simulink model "lin_model_PI_MRAC_Sim_CASE1_L1"  (Simulink 7.7)
settings: Solver=ode45  StartTime=0.0  StopTime=TIME  RelTol=1e-3  AbsTol=1e-6
values from neighbouring files (symbols this model uses):
  Am = AA - BB*Kr    [lin_model_LQR.m]    (also in lin_model_PI_MRAC_CASE1.m = Ar-BB*Kr; lin_model_PI_MRAC_CASE1_L1.m = Ar-BB*Kr)
  Ar = Ar_cruise    [parameter.m]
  BB = B_cruise    [parameter.m]
  bm = -(CC*inv(Am))\eye(11)    [lin_model_PI_MRAC_CASE1.m]    (also in lin_model_PI_MRAC_CASE1_L1.m)
  gamma = rho*c_cr*a_cr*(r_cr)^4/Icr    (= 0.431761992187)    [beta_crS.m]    (also in heli_parameter.m = 5.40374741035; lin_model_PI_MRAC_CASE1.m = 1000000; lin_model_PI_MRAC_CASE1_L1.m = 10000; parameter.m = 5.40374741035)
  noise = 0.1    [lin_model_PI_MRAC_CASE1_L1.m]
  omega = 10    [lin_model_PI_MRAC_CASE1_L1.m]
  pulse = 1    [lin_model_PI_MRAC_CASE1_L1.m]
  tau = 0.01    [lin_model_PI_MRAC_CASE1_L1.m]
  Theta_a = AA-Ar    [parameter.m]
  theta_hat0 = eye(11)    [lin_model_PI_MRAC_CASE1.m]    (also in lin_model_PI_MRAC_CASE1_L1.m)
  unmodeled = 1    [lin_model_PI_MRAC_CASE1_L1.m]
  x0 = [0;0;0;0]    [beta_crS.m]    (also in flapping.m = []; flappingthrust.m = []; lin_flapping.m = []; lin_model_LQR.m = [3 3 3 0 0 0 0 0 0 0 0]')
  x_hat0 = x0    [lin_model_PI_MRAC_CASE1.m]    (also in lin_model_PI_MRAC_CASE1_L1.m)
undefined symbols (not defined in the file or in its folder): Kr
libraries: simulink x3, commnoisgen2 x1
settings Model: Creator=Li  LastModifiedBy=Li
settings DataIOCC: LimitDataPoints=off  SaveFormat=Structure
settings DebuggingCC: SolverPrmCheckMsg=none

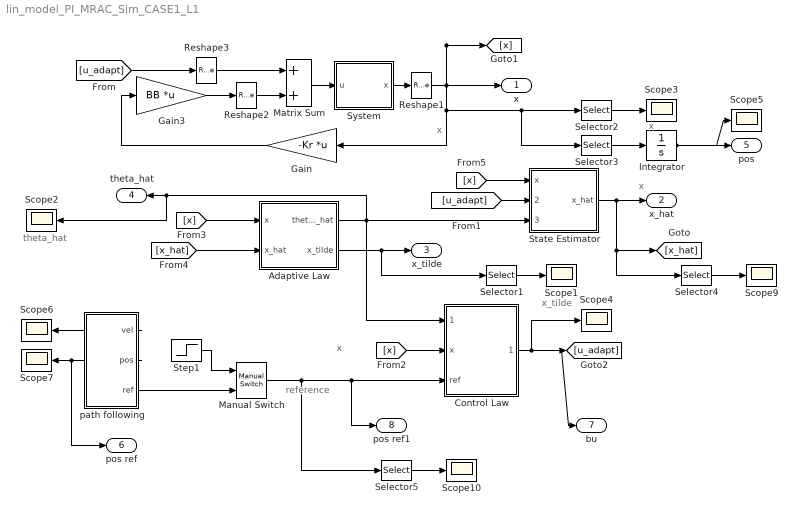
== system lin_model_PI_MRAC_Sim_CASE1_L1 ==
  note: x
  note: x
  note: reference
  note: theta_hat
  note: x_tilde
  note: x
  note: x
  Adaptive Law : Subsystem
  Control Law : Subsystem
  Gain : Gain  Gain=-Kr  Multiplication=Matrix(K*u) (u vector)
  Gain3 : Gain  Gain=BB  Multiplication=Matrix(K*u) (u vector)
  Integrator : Integrator
  Manual Switch : simulink/Signal Routing/Manual Switch  SystemSampleTime=-1  sw=0  action=0  varsize=off
  Matrix Sum : Sum
  Reshape1 : Reshape  OutputDimensionality=Column vector (2-D)
  Reshape2 : Reshape  OutputDimensionality=Column vector (2-D)
  Reshape3 : Reshape  OutputDimensionality=Column vector (2-D)
  Scope{1..7,9..10} (9 alike) : Scope
      Scope1 settings: TimeRange=3  YMin=-3e+007  YMax=2.5e+006
      Scope10 settings: TimeRange=10  YMin=-15  YMax=15  SaveName=ScopeData9
      Scope2 settings: TimeRange=20  YMin=-1  YMax=1
      Scope3 settings: TimeRange=10  YMin=-1400  YMax=0  SaveName=ScopeData2
      Scope4 settings: TimeRange=20  YMin=-150  YMax=300  SaveName=ScopeData3
      Scope5 settings: TimeRange=10  YMin=-3000  YMax=3000  SaveName=ScopeData4
      Scope6 settings: TimeRange=10  YMin=-3000  YMax=3000  SaveName=ScopeData5
      Scope7 settings: TimeRange=10  YMin=-3000  YMax=3000  SaveName=ScopeData6
      Scope9 settings: TimeRange=10  YMin=-15  YMax=17.5  SaveName=ScopeData8
  Selector1 : Selector  InputPortWidth=11  IndexOptions=Index vector (dialog)  Indices=[1 2 3 4 5]  OutputSizes=1
  Selector{2..5} (4 alike) : Selector  InputPortWidth=11  IndexOptions=Index vector (dialog)  Indices=[1 2 3]  OutputSizes=1
  State Estimator : Subsystem
  Step1 : Step  Time=5  Before=[15 0 0 0 0 0 0 0 0 0 0]'  After=[10 -5 2 0 0 0 0 0 0 0 0]'  SampleTime=0
  System : Subsystem
  path following : Subsystem
  x : Outport
  x_hat : Outport  Port=2
  x_tilde : Outport  Port=3
  theta_hat : Outport  Port=4
  pos : Outport  Port=5
  pos ref : Outport  Port=6
  bu : Outport  Port=7
  pos ref1 : Outport  Port=8
  wires:
  Matrix Sum/1 -> System/1(u)
  State Estimator/1(x_hat) -> x_hat/1, [x_hat], Selector4/1
  [u_adapt] -> State Estimator/2(u_adapt)
  Gain/1 -> Gain3/1
  [x] -> Adaptive Law/1(x)
  [x_hat] -> Adaptive Law/2(x_hat)
  Adaptive Law/1(theta_hat) -> State Estimator/3(theta_hat), Control Law/1(theta_hat), theta_hat/1, Scope2/1
  Control Law/1(u_adap) -> [u_adapt], Scope4/1, bu/1
  Manual Switch/1 -> Control Law/3(ref), pos ref1/1, Selector5/1
  System/1(x) -> Reshape1/1
  Reshape1/1 -> x/1, [x], Gain/1, Selector2/1, Selector3/1
  Gain3/1 -> Reshape2/1
  Reshape2/1 -> Matrix Sum/2
  [u_adapt] -> Reshape3/1
  Reshape3/1 -> Matrix Sum/1
  Selector1/1 -> Scope1/1
  Adaptive Law/2(x_tilde) -> x_tilde/1, Selector1/1
  Selector2/1 -> Scope3/1
  [x] -> Control Law/2(x)
  [x] -> State Estimator/1(x)
  Selector3/1 -> Integrator/1
  Integrator/1 -> pos/1, Scope5/1
  path following/3(ref) -> Manual Switch/2
  path following/1(vel) -> Scope6/1
  path following/2(pos) -> Scope7/1, pos ref/1
  Selector4/1 -> Scope9/1
  Selector5/1 -> Scope10/1
  Step1/1 -> Manual Switch/1

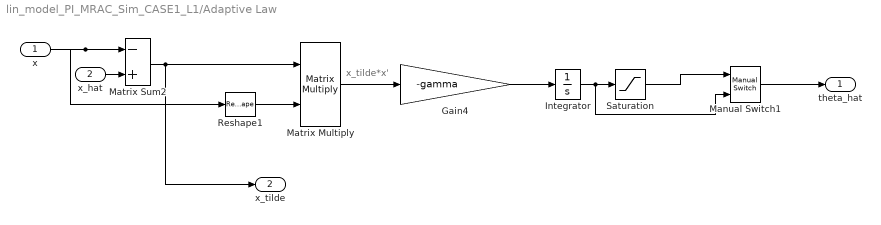
== system lin_model_PI_MRAC_Sim_CASE1_L1/Adaptive Law ==
  note: x_tilde*x'
  x : Inport
  x_hat : Inport  Port=2
  Gain4 : Gain  Gain=-gamma
  Integrator : Integrator  InitialCondition=theta_hat0
  Manual Switch1 : simulink/Signal Routing/Manual Switch  SystemSampleTime=-1  sw=0  action=0  varsize=off
  Matrix Sum2 : Sum  Inputs=-+
  Matrix Multiply : Product  Multiplication=Matrix(*)
  Reshape1 : Reshape  OutputDimensionality=Row vector (2-D)
  Saturation : Saturate  UpperLimit=50  LowerLimit=-50
  theta_hat : Outport
  x_tilde : Outport  Port=2
  wires:
  Matrix Sum2/1 -> Matrix Multiply/1, x_tilde/1
  Reshape1/1 -> Matrix Multiply/2
  Matrix Multiply/1 -> Gain4/1
  x/1 -> Matrix Sum2/1, Reshape1/1
  x_hat/1 -> Matrix Sum2/2
  Gain4/1 -> Integrator/1
  Integrator/1 -> Manual Switch1/2, Saturation/1
  Manual Switch1/1 -> theta_hat/1
  Saturation/1 -> Manual Switch1/1

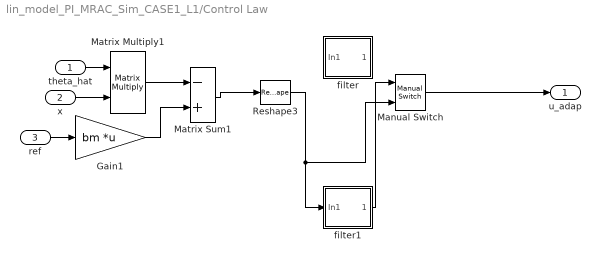
== system lin_model_PI_MRAC_Sim_CASE1_L1/Control Law ==
  theta_hat : Inport
  x : Inport  Port=2
  ref : Inport  Port=3
  Gain1 : Gain  Gain=bm  Multiplication=Matrix(K*u) (u vector)
  Manual Switch : simulink/Signal Routing/Manual Switch  SystemSampleTime=-1  sw=1  action=0  varsize=off
  Matrix Sum1 : Sum  Inputs=-+
  Matrix Multiply1 : Product  Multiplication=Matrix(*)
  Reshape3 : Reshape  OutputDimensionality=Column vector (2-D)
  filter : Subsystem
  filter1 : Subsystem
  u_adap : Outport
  wires:
  Matrix Multiply1/1 -> Matrix Sum1/1
  x/1 -> Matrix Multiply1/2
  theta_hat/1 -> Matrix Multiply1/1
  ref/1 -> Gain1/1
  Matrix Sum1/1 -> Reshape3/1
  Reshape3/1 -> Manual Switch/2, filter1/1(In1)
  Gain1/1 -> Matrix Sum1/2
  Manual Switch/1 -> u_adap/1
  filter1/1(Out1) -> Manual Switch/1

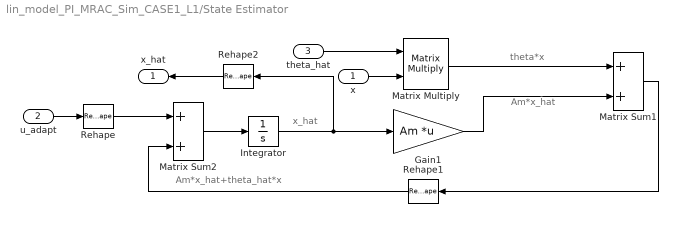
== system lin_model_PI_MRAC_Sim_CASE1_L1/State Estimator ==
  note: x_hat
  note: theta*x
  note: Am*x_hat
  note: Am*x_hat+theta_hat*x
  x : Inport
  u_adapt : Inport  Port=2
  theta_hat : Inport  Port=3
  Gain1 : Gain  Gain=Am  Multiplication=Matrix(K*u) (u vector)
  Integrator : Integrator  InitialCondition=x_hat0
  Matrix Sum1 : Sum
  Matrix Sum2 : Sum
  Matrix Multiply : Product  Multiplication=Matrix(*)
  Rehape : Reshape  OutputDimensionality=Column vector (2-D)
  Rehape1 : Reshape  OutputDimensionality=Column vector (2-D)
  Rehape2 : Reshape  OutputDimensionality=Column vector (2-D)
  x_hat : Outport
  wires:
  theta_hat/1 -> Matrix Multiply/1
  Integrator/1 -> Gain1/1, Rehape2/1
  Matrix Multiply/1 -> Matrix Sum1/1
  Gain1/1 -> Matrix Sum1/2
  Matrix Sum2/1 -> Integrator/1
  x/1 -> Matrix Multiply/2
  Rehape/1 -> Matrix Sum2/1
  u_adapt/1 -> Rehape/1
  Matrix Sum1/1 -> Rehape1/1
  Rehape1/1 -> Matrix Sum2/2
  Rehape2/1 -> x_hat/1

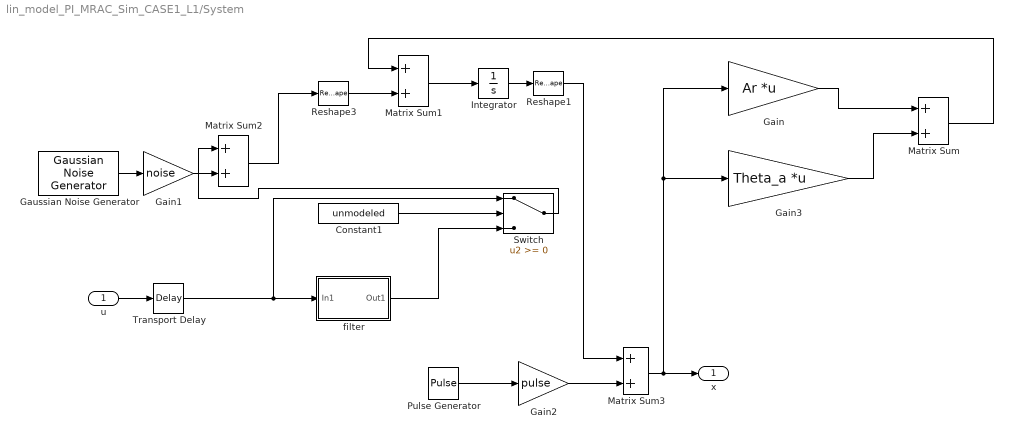
== system lin_model_PI_MRAC_Sim_CASE1_L1/System ==
  u : Inport
  Constant1 : Constant  Value=unmodeled
  Gain : Gain  Gain=Ar  Multiplication=Matrix(K*u) (u vector)
  Gain1 : Gain  Gain=noise
  Gain2 : Gain  Gain=pulse
  Gain3 : Gain  Gain=Theta_a  Multiplication=Matrix(K*u) (u vector)
  Gaussian Noise Generator : commnoisgen2/Gaussian Noise Generator  SystemSampleTime=-1  m=0  d=1*ones(11,1)  s=41  Ts=1  frameBased=off  sampPerFrame=1  orient=off  outDataType=double
  Integrator : Integrator  InitialCondition=x0
  Matrix Sum{,1..3} (4 alike) : Sum
  Pulse Generator : DiscretePulseGenerator  PulseType=Time based  Amplitude=[1 0 0 0 0 0 0 0 0 0 0];  Period=7  PulseWidth=2  PhaseDelay=3
  Reshape1 : Reshape  OutputDimensionality=Column vector (2-D)
  Reshape3 : Reshape  OutputDimensionality=Column vector (2-D)
  Switch : Switch
  Transport Delay : TransportDelay  DelayTime=tau
  filter : Subsystem
  x : Outport
  wires:
  Gain/1 -> Matrix Sum/1
  Gain3/1 -> Matrix Sum/2
  Matrix Sum1/1 -> Integrator/1
  Matrix Sum/1 -> Matrix Sum1/1
  Integrator/1 -> Reshape1/1
  Reshape1/1 -> Matrix Sum3/1
  Reshape3/1 -> Matrix Sum1/2
  Constant1/1 -> Switch/2
  Matrix Sum2/1 -> Reshape3/1
  Switch/1 -> Matrix Sum2/1
  u/1 -> Transport Delay/1
  Transport Delay/1 -> Switch/1, filter/1(In1)
  Gaussian Noise Generator/1 -> Gain1/1
  Gain1/1 -> Matrix Sum2/2
  filter/1(Out1) -> Switch/3
  Matrix Sum3/1 -> x/1, Gain/1, Gain3/1
  Pulse Generator/1 -> Gain2/1
  Gain2/1 -> Matrix Sum3/2

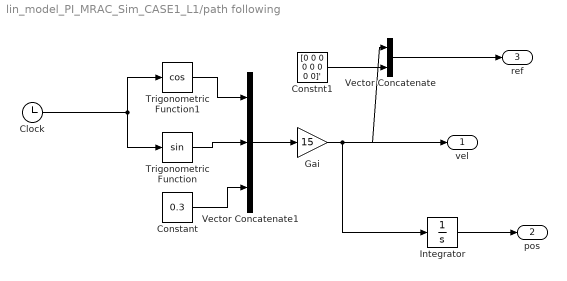
== system lin_model_PI_MRAC_Sim_CASE1_L1/path following ==
  Clock : Clock
      settings: Decimation=10
  Constant : Constant  Value=0.3
  Constnt1 : Constant  Value=[0 0 0 0 0 0 0 0]'
  Gai : Gain  Gain=15
  Integrator : Integrator
  Trigonometric Function : Trigonometry
  Trigonometric Function1 : Trigonometry  Operator=cos
  Vector Concatenate : Concatenate  Mode=Vector
  Vector Concatenate1 : Concatenate  NumInputs=3  Mode=Vector
  vel : Outport
  pos : Outport  Port=2
  ref : Outport  Port=3
  wires:
  Clock/1 -> Trigonometric Function/1, Trigonometric Function1/1
  Trigonometric Function1/1 -> Vector Concatenate1/1
  Trigonometric Function/1 -> Vector Concatenate1/2
  Constant/1 -> Vector Concatenate1/3
  Vector Concatenate1/1 -> Gai/1
  Gai/1 -> Integrator/1, Vector Concatenate/1, vel/1
  Integrator/1 -> pos/1
  Constnt1/1 -> Vector Concatenate/2
  Vector Concatenate/1 -> ref/1

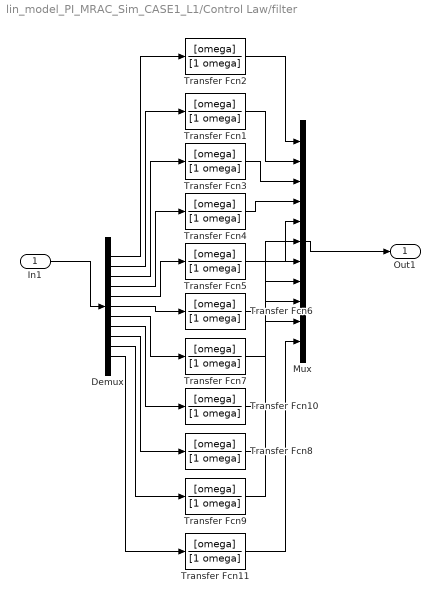
== system lin_model_PI_MRAC_Sim_CASE1_L1/Control Law/filter ==
  In1 : Inport
  Demux : Demux  Outputs=11
  Mux : Mux  Inputs=11
  Transfer Fcn1 : TransferFcn  RequirementInfo={} %GIDa_1588be67_b809_4f16_8238_c529f8c71181  Numerator=[omega]  Denominator=[1 omega]
  Transfer Fcn10 : TransferFcn  RequirementInfo={} %GIDa_86af2edf_03e9_4a24_9dc1_ce3410ca81b3  Numerator=[omega]  Denominator=[1 omega]
  Transfer Fcn11 : TransferFcn  RequirementInfo={} %GIDa_81acbab7_09e6_45bb_a54d_a731545e4437  Numerator=[omega]  Denominator=[1 omega]
  Transfer Fcn2 : TransferFcn  RequirementInfo={} %GIDa_ef890eef_aa48_4047_8ef5_145ca425c186  Numerator=[omega]  Denominator=[1 omega]
  Transfer Fcn3 : TransferFcn  RequirementInfo={} %GIDa_2223c891_cefd_426d_9500_0a238d8c2f6d  Numerator=[omega]  Denominator=[1 omega]
  Transfer Fcn4 : TransferFcn  RequirementInfo={} %GIDa_1824c089_893d_419d_8145_f79434dd5c18  Numerator=[omega]  Denominator=[1 omega]
  Transfer Fcn5 : TransferFcn  RequirementInfo={} %GIDa_d6696dcf_ee0c_4ba6_8e67_8290c8b1e36c  Numerator=[omega]  Denominator=[1 omega]
  Transfer Fcn6 : TransferFcn  RequirementInfo={} %GIDa_74c39ed2_1dac_4ad6_9ded_3c413e9dd9f0  Numerator=[omega]  Denominator=[1 omega]
  Transfer Fcn7 : TransferFcn  RequirementInfo={} %GIDa_f655826e_06f8_4ed3_9a30_9fafda06148a  Numerator=[omega]  Denominator=[1 omega]
  Transfer Fcn8 : TransferFcn  RequirementInfo={} %GIDa_e198e039_0c18_4aae_a29d_3d26360fa2df  Numerator=[omega]  Denominator=[1 omega]
  Transfer Fcn9 : TransferFcn  RequirementInfo={} %GIDa_ce4bca28_29e3_49d8_b971_70edd09c1024  Numerator=[omega]  Denominator=[1 omega]
  Out1 : Outport
  wires:
  In1/1 -> Demux/1
  Demux/1 -> Transfer Fcn2/1
  Demux/2 -> Transfer Fcn1/1
  Demux/3 -> Transfer Fcn3/1
  Demux/4 -> Transfer Fcn4/1
  Demux/5 -> Transfer Fcn5/1
  Demux/6 -> Transfer Fcn6/1
  Demux/7 -> Transfer Fcn7/1
  Demux/8 -> Transfer Fcn10/1
  Demux/9 -> Transfer Fcn8/1
  Demux/10 -> Transfer Fcn9/1
  Mux/1 -> Out1/1
  Transfer Fcn2/1 -> Mux/1
  Transfer Fcn1/1 -> Mux/2
  Transfer Fcn3/1 -> Mux/3
  Transfer Fcn4/1 -> Mux/4
  Transfer Fcn5/1 -> Mux/5
  Transfer Fcn6/1 -> Mux/6
  Transfer Fcn7/1 -> Mux/7
  Transfer Fcn10/1 -> Mux/8
  Transfer Fcn8/1 -> Mux/9
  Transfer Fcn9/1 -> Mux/10
  Transfer Fcn11/1 -> Mux/11
  Demux/11 -> Transfer Fcn11/1

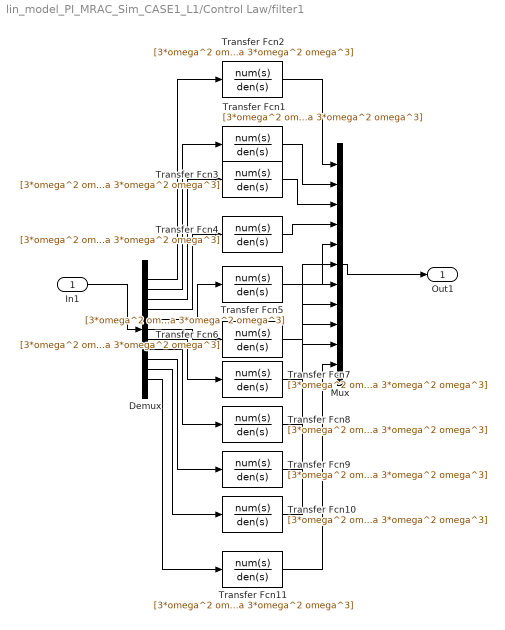
== system lin_model_PI_MRAC_Sim_CASE1_L1/Control Law/filter1 ==
  In1 : Inport
  Demux : Demux  Outputs=11
  Mux : Mux  Inputs=11
  Transfer Fcn1 : TransferFcn  RequirementInfo={} %GIDa_6649f815_cf1e_4a6d_880e_da1b620a08ec  Numerator=[3*omega^2 omega^3]  Denominator=[1 3*omega 3*omega^2 omega^3]
  Transfer Fcn10 : TransferFcn  RequirementInfo={} %GIDa_10410983_3204_4eb8_9c86_7dd871c6b653  Numerator=[3*omega^2 omega^3]  Denominator=[1 3*omega 3*omega^2 omega^3]
  Transfer Fcn11 : TransferFcn  RequirementInfo={} %GIDa_a97dd7c5_f6e2_4bba_b584_93a15a1f4f7b  Numerator=[3*omega^2 omega^3]  Denominator=[1 3*omega 3*omega^2 omega^3]
  Transfer Fcn2 : TransferFcn  RequirementInfo={} %GIDa_c2ce4450_f1b2_41af_aca2_5a2fc8095075  Numerator=[3*omega^2 omega^3]  Denominator=[1 3*omega 3*omega^2 omega^3]
  Transfer Fcn3 : TransferFcn  RequirementInfo={} %GIDa_dce21328_ab85_4136_a047_f0b12e1c45a6  Numerator=[3*omega^2 omega^3]  Denominator=[1 3*omega 3*omega^2 omega^3]
  Transfer Fcn4 : TransferFcn  RequirementInfo={} %GIDa_409c4cfe_4b8e_4925_8bf3_b829eac12b94  Numerator=[3*omega^2 omega^3]  Denominator=[1 3*omega 3*omega^2 omega^3]
  Transfer Fcn5 : TransferFcn  RequirementInfo={} %GIDa_397d628d_3faa_4950_bae8_37d8c5b8f5a0  Numerator=[3*omega^2 omega^3]  Denominator=[1 3*omega 3*omega^2 omega^3]
  Transfer Fcn6 : TransferFcn  RequirementInfo={} %GIDa_c7b56593_de39_4929_bff3_f278f6b26593  Numerator=[3*omega^2 omega^3]  Denominator=[1 3*omega 3*omega^2 omega^3]
  Transfer Fcn7 : TransferFcn  RequirementInfo={} %GIDa_b7d18214_1dfe_4961_a910_ed0f44c32057  Numerator=[3*omega^2 omega^3]  Denominator=[1 3*omega 3*omega^2 omega^3]
  Transfer Fcn8 : TransferFcn  RequirementInfo={} %GIDa_796c0fd5_bb02_4140_a290_e55335a61e28  Numerator=[3*omega^2 omega^3]  Denominator=[1 3*omega 3*omega^2 omega^3]
  Transfer Fcn9 : TransferFcn  RequirementInfo={} %GIDa_ad3b18aa_da55_4a73_89f5_b050e907d0ca  Numerator=[3*omega^2 omega^3]  Denominator=[1 3*omega 3*omega^2 omega^3]
  Out1 : Outport
  wires:
  In1/1 -> Demux/1
  Demux/1 -> Transfer Fcn2/1
  Demux/2 -> Transfer Fcn1/1
  Demux/3 -> Transfer Fcn3/1
  Demux/4 -> Transfer Fcn4/1
  Demux/5 -> Transfer Fcn5/1
  Demux/6 -> Transfer Fcn6/1
  Demux/7 -> Transfer Fcn7/1
  Demux/8 -> Transfer Fcn8/1
  Demux/9 -> Transfer Fcn9/1
  Demux/10 -> Transfer Fcn10/1
  Mux/1 -> Out1/1
  Transfer Fcn2/1 -> Mux/1
  Transfer Fcn1/1 -> Mux/2
  Transfer Fcn3/1 -> Mux/3
  Transfer Fcn4/1 -> Mux/4
  Transfer Fcn5/1 -> Mux/5
  Transfer Fcn6/1 -> Mux/6
  Transfer Fcn7/1 -> Mux/7
  Transfer Fcn8/1 -> Mux/8
  Transfer Fcn9/1 -> Mux/9
  Transfer Fcn10/1 -> Mux/10
  Transfer Fcn11/1 -> Mux/11
  Demux/11 -> Transfer Fcn11/1

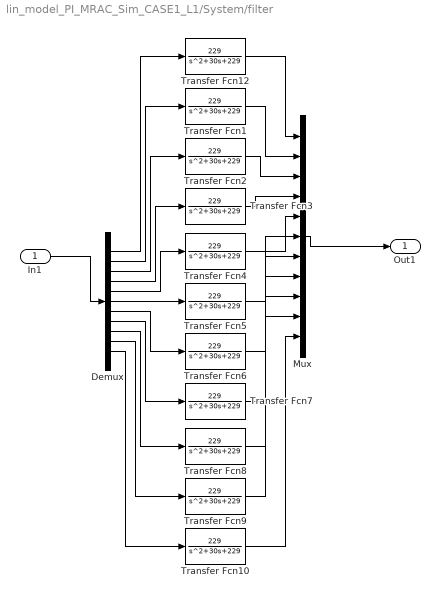
== system lin_model_PI_MRAC_Sim_CASE1_L1/System/filter ==
  In1 : Inport
  Demux : Demux  Outputs=11
  Mux : Mux  Inputs=11
  Transfer Fcn{1..10,12} (11 alike) : TransferFcn  Numerator=[229]  Denominator=[1 30 229]
  Out1 : Outport
  wires:
  In1/1 -> Demux/1
  Demux/1 -> Transfer Fcn12/1
  Demux/2 -> Transfer Fcn1/1
  Demux/3 -> Transfer Fcn2/1
  Demux/4 -> Transfer Fcn3/1
  Demux/5 -> Transfer Fcn4/1
  Demux/6 -> Transfer Fcn5/1
  Demux/7 -> Transfer Fcn6/1
  Demux/8 -> Transfer Fcn7/1
  Demux/9 -> Transfer Fcn8/1
  Demux/10 -> Transfer Fcn9/1
  Mux/1 -> Out1/1
  Transfer Fcn12/1 -> Mux/1
  Transfer Fcn1/1 -> Mux/2
  Transfer Fcn2/1 -> Mux/3
  Transfer Fcn3/1 -> Mux/4
  Transfer Fcn4/1 -> Mux/5
  Transfer Fcn5/1 -> Mux/6
  Transfer Fcn6/1 -> Mux/7
  Transfer Fcn7/1 -> Mux/8
  Transfer Fcn8/1 -> Mux/9
  Transfer Fcn9/1 -> Mux/10
  Transfer Fcn10/1 -> Mux/11
  Demux/11 -> Transfer Fcn10/1
